simulink model "poleplace_sfb_luenburg_roo"  (Simulink 7.5)
settings: Solver=ode4  StartTime=0.0  StopTime=6  FixedStep=0.05  RelTol=1e-3
PreLoadFcn:
  | poleplace_sfb_luenburg_roo_param
values from neighbouring files (symbols this model uses):
  A = [0  -20.6; 1 0],    [poleplace_luenburg_foo_param.m]    (also in poleplace_luenburg_roo_param.m = [0  1  0; 0  0  1; 0  0  0],; poleplace_sfb_luenburg_foo_param.m = [0  1; 0  -5],; poleplace_sfb_luenburg_roo_param.m = [0  1  0; 0  0  1; -6  -11  -6],)
  AA = A11 - G*A21,    [poleplace_luenburg_roo_param.m]    (also in poleplace_sfb_luenburg_roo_param.m = Abb - G*Aab,)
  B = [0; 1],    [poleplace_luenburg_foo_param.m]    (also in poleplace_luenburg_roo_param.m = [0; 0; 1],; poleplace_sfb_luenburg_foo_param.m = [0; 100],; poleplace_sfb_luenburg_roo_param.m = [0; 0; 1],)
  BB = B_1 - G*B_2,    [poleplace_luenburg_roo_param.m]    (also in poleplace_sfb_luenburg_roo_param.m = Bb - G*Ba,)
  C = [0 1],    [poleplace_luenburg_foo_param.m]    (also in poleplace_luenburg_roo_param.m = [1 0 0],; poleplace_sfb_luenburg_foo_param.m = [1 0],; poleplace_sfb_luenburg_roo_param.m = [1 0 0],)
  CC = [zeros(m, n-m); eye(n-m)],    [poleplace_sfb_luenburg_roo_param.m]
  DD = [eye(m); G],    [poleplace_sfb_luenburg_roo_param.m]
  GG = (A11 - G*A21)*G + (A12-G*A22),    [poleplace_luenburg_roo_param.m]    (also in poleplace_sfb_luenburg_roo_param.m = (Abb - G*Aab)*G + (Aba - G*Aaa),)
  K = acker(A, B, p),    [poleplace_sfb_luenburg_foo_param.m]    (also in poleplace_sfb_luenburg_roo_param.m = acker(A, B, pole_ctrl_desired),)
libraries: simulink x1
settings Model: Creator=Huiliang  LastModifiedBy=Dell
settings OptimizationCC: InitFltsAndDblsToZero=on
settings DebuggingCC: SaveWithParameterizedLinksMsg=none  StrictBusMsg=Warning
settings GRTTargetCC: TargetFcnLib=ansi_tfl_tmw.mat

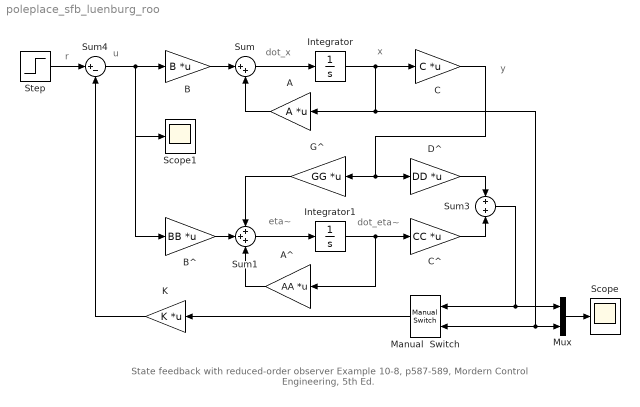
== system poleplace_sfb_luenburg_roo ==
  note: x
  note: dot_x
  note: y
  note: u
  note: eta~
  note: dot_eta~
  note: r
  note: State feedback with reduced-order observer
      | Example 10-8, p587-589, Mordern Control Engineering, 5th Ed.
  A : Gain  Gain=A  Multiplication=Matrix(K*u)  ParameterDataType=sfix(16)  ParameterScaling=2^0  OutDataType=sfix(16)  OutScaling=2^0
  A^ : Gain  Gain=AA  Multiplication=Matrix(K*u)  ParameterDataType=sfix(16)  ParameterScaling=2^0  OutDataType=sfix(16)  OutScaling=2^0
  B : Gain  Gain=B  Multiplication=Matrix(K*u)  ParameterDataType=sfix(16)  ParameterScaling=2^0  OutDataType=sfix(16)  OutScaling=2^0
  B^ : Gain  Gain=BB  Multiplication=Matrix(K*u)  ParameterDataType=sfix(16)  ParameterScaling=2^0  OutDataType=sfix(16)  OutScaling=2^0
  C : Gain  Gain=C  Multiplication=Matrix(K*u)  ParameterDataType=sfix(16)  ParameterScaling=2^0  OutDataType=sfix(16)  OutScaling=2^0
  C^ : Gain  Gain=CC  Multiplication=Matrix(K*u)  ParameterDataType=sfix(16)  ParameterScaling=2^0  OutDataType=sfix(16)  OutScaling=2^0
  D^ : Gain  Gain=DD  Multiplication=Matrix(K*u)  ParameterDataType=sfix(16)  ParameterScaling=2^0  OutDataType=sfix(16)  OutScaling=2^0
  G^ : Gain  Gain=GG  Multiplication=Matrix(K*u)  ParameterDataType=sfix(16)  ParameterScaling=2^0  OutDataType=sfix(16)  OutScaling=2^0
  Integrator : Integrator  InitialCondition="[0;   0.01;  0 ]"
  Integrator1 : Integrator  InitialCondition="[0;    0]"
  K : Gain  Gain=K  Multiplication=Matrix(K*u)  ParameterDataType=sfix(16)  ParameterScaling=2^0  OutDataType=sfix(16)  OutScaling=2^0
  Manual  Switch : simulink/Signal Routing/Manual Switch  SystemSampleTime=-1  sw=1  action=0  varsize=off
  Mux : Mux  Inputs=2
  Scope : Scope
      settings: TimeRange=6  YMin=-0.04  YMax=0.04
  Scope1 : Scope
      settings: TimeRange=6  YMin=-1  YMax=1
  Step : Step  Time=3  SampleTime=0
  Sum : Sum  Inputs=|++  OutDataType=sfix(16)  OutScaling=2^0
  Sum1 : Sum  Inputs=+++  OutDataType=sfix(16)  OutScaling=2^0
  Sum3 : Sum  Inputs=+|+  OutDataType=sfix(16)  OutScaling=2^0
  Sum4 : Sum  Inputs=|+-  OutDataType=sfix(16)  OutScaling=2^0
  wires:
  Integrator/1 -> C/1, A/1, Manual  Switch/2, Mux/2
  Sum/1 -> Integrator/1
  B/1 -> Sum/1
  Step/1 -> Sum4/1
  K/1 -> Sum4/2
  Sum4/1 -> B/1, B^/1, Scope1/1
  C/1 -> G^/1, D^/1
  B^/1 -> Sum1/2
  Sum1/1 -> Integrator1/1
  Integrator1/1 -> C^/1, A^/1
  Mux/1 -> Scope/1
  D^/1 -> Sum3/1
  C^/1 -> Sum3/2
  Manual  Switch/1 -> K/1
  G^/1 -> Sum1/1
  A^/1 -> Sum1/3
  A/1 -> Sum/2
  Sum3/1 -> Manual  Switch/1, Mux/1
